simulink model "Irrigation_Control_System_R2020a"  (R2023b)
settings: Solver=VariableStepAuto  StartTime=0.0  StopTime=10.0  MaxStep=1e-3  RelTol=1e-3
libraries: simulink x1
settings Model: Creator=hp  LastModifiedBy=hp
settings SolverCC: AlgebraicLoopSolver=TrustRegion

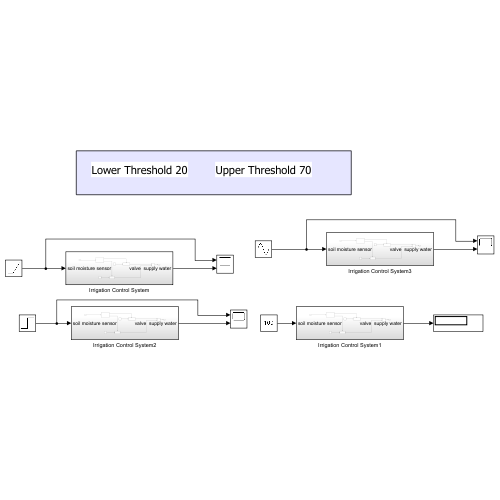
[thumbnail: Simulink's stored preview of the top-level diagram]
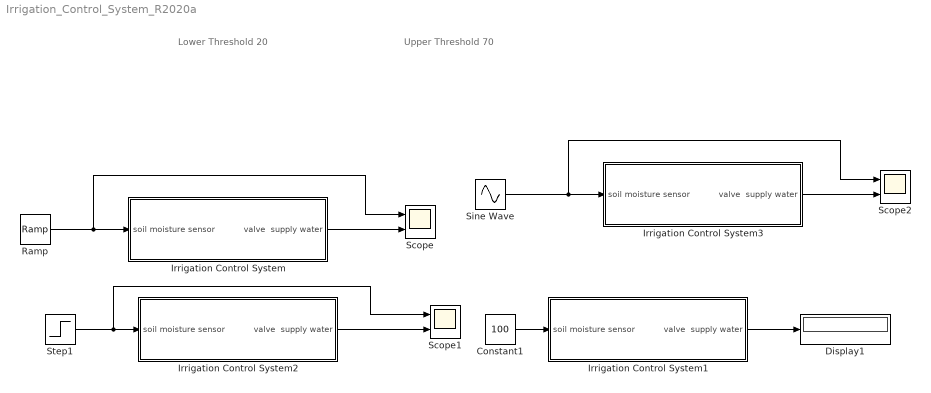
== system Irrigation_Control_System_R2020a ==
  note: Lower Threshold 20
  note: Upper Threshold 70
  Constant1 : Constant  Value=100
  Display1 : Display
  Irrigation Control System : Subsystem
  Irrigation Control System1 : Subsystem
  Irrigation Control System2 : Subsystem
  Irrigation Control System3 : Subsystem
  Ramp : simulink/Sources/Ramp  slope=1  start=0  InitialOutput=15
  Scope : Scope  NumInputPorts=2
  Scope1 : Scope  NumInputPorts=2
  Scope2 : Scope  NumInputPorts=2
  Sine Wave : Sin  Amplitude=50  SampleTime=0
  Step1 : Step  Before=5  After=70  SampleTime=0
  wires:
  Irrigation Control System1/1(valve  supply water) -> Display1/1
  Constant1/1 -> Irrigation Control System1/1(soil moisture sensor)
  Irrigation Control System/1(valve  supply water) -> Scope/2
  Ramp/1 -> Scope/1, Irrigation Control System/1(soil moisture sensor)
  Step1/1 -> Scope1/1, Irrigation Control System2/1(soil moisture sensor)
  Irrigation Control System2/1(valve  supply water) -> Scope1/2
  Sine Wave/1 -> Irrigation Control System3/1(soil moisture sensor), Scope2/1
  Irrigation Control System3/1(valve  supply water) -> Scope2/2

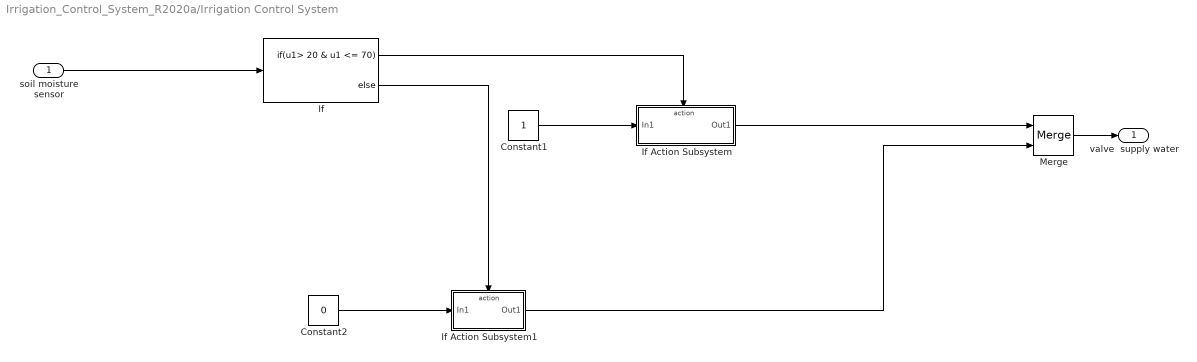
== system Irrigation_Control_System_R2020a/Irrigation Control System ==
  soil moisture sensor : Inport
  Constant1 : Constant
  Constant2 : Constant  Value=0
  If : If  IfExpression=u1> 20 & u1 <= 70
  If Action Subsystem : Subsystem  TreatAsAtomicUnit=on
  If Action Subsystem1 : Subsystem  TreatAsAtomicUnit=on
  Merge : Merge
  valve  supply water : Outport
  wires:
  If Action Subsystem/1(Out1) -> Merge/1
  Constant2/1 -> If Action Subsystem1/1(In1)
  If/2 -> If Action Subsystem1/Action
  If/1 -> If Action Subsystem/Action
  soil moisture sensor/1 -> If/1
  Merge/1 -> valve  supply water/1
  Constant1/1 -> If Action Subsystem/1(In1)
  If Action Subsystem1/1(Out1) -> Merge/2

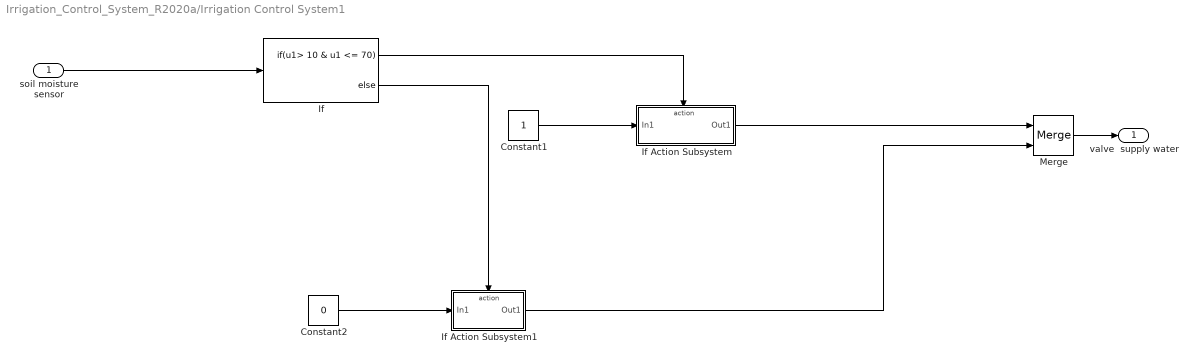
== system Irrigation_Control_System_R2020a/Irrigation Control System1 ==
  soil moisture sensor : Inport
  Constant1 : Constant
  Constant2 : Constant  Value=0
  If : If  IfExpression=u1> 10 & u1 <= 70
  If Action Subsystem : Subsystem  TreatAsAtomicUnit=on
  If Action Subsystem1 : Subsystem  TreatAsAtomicUnit=on
  Merge : Merge
  valve  supply water : Outport
  wires:
  If Action Subsystem1/1(Out1) -> Merge/2
  Constant1/1 -> If Action Subsystem/1(In1)
  Merge/1 -> valve  supply water/1
  soil moisture sensor/1 -> If/1
  If/1 -> If Action Subsystem/Action
  If/2 -> If Action Subsystem1/Action
  Constant2/1 -> If Action Subsystem1/1(In1)
  If Action Subsystem/1(Out1) -> Merge/1

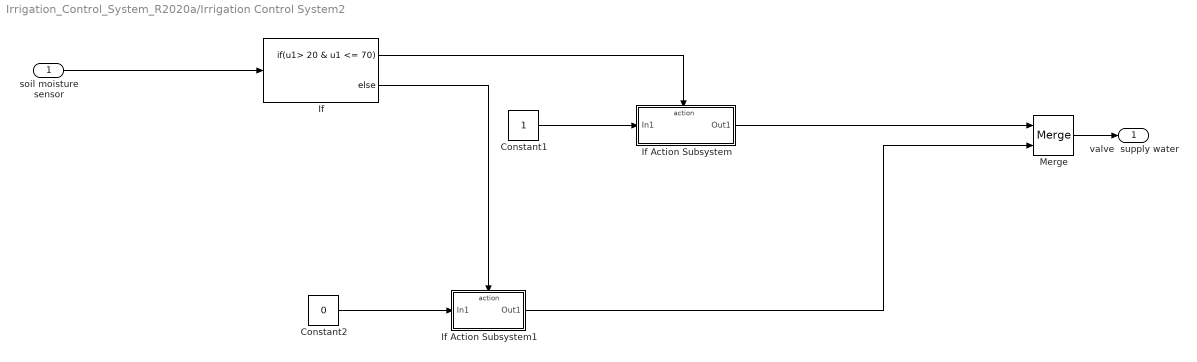
== system Irrigation_Control_System_R2020a/Irrigation Control System2 ==
  soil moisture sensor : Inport
  Constant1 : Constant
  Constant2 : Constant  Value=0
  If : If  IfExpression=u1> 20 & u1 <= 70
  If Action Subsystem : Subsystem  TreatAsAtomicUnit=on
  If Action Subsystem1 : Subsystem  TreatAsAtomicUnit=on
  Merge : Merge
  valve  supply water : Outport
  wires:
  If Action Subsystem1/1(Out1) -> Merge/2
  Constant1/1 -> If Action Subsystem/1(In1)
  Merge/1 -> valve  supply water/1
  soil moisture sensor/1 -> If/1
  If/1 -> If Action Subsystem/Action
  If/2 -> If Action Subsystem1/Action
  Constant2/1 -> If Action Subsystem1/1(In1)
  If Action Subsystem/1(Out1) -> Merge/1

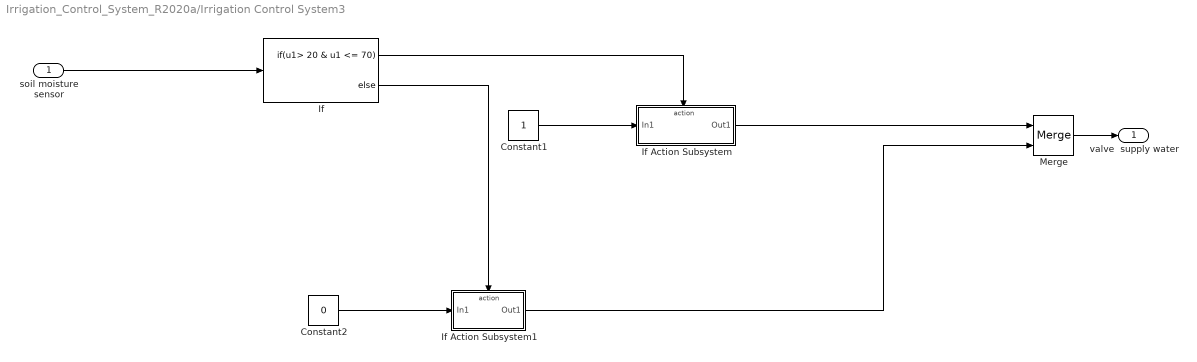
== system Irrigation_Control_System_R2020a/Irrigation Control System3 ==
  soil moisture sensor : Inport
  Constant1 : Constant
  Constant2 : Constant  Value=0
  If : If  IfExpression=u1> 20 & u1 <= 70
  If Action Subsystem : Subsystem  TreatAsAtomicUnit=on
  If Action Subsystem1 : Subsystem  TreatAsAtomicUnit=on
  Merge : Merge
  valve  supply water : Outport
  wires:
  If Action Subsystem1/1(Out1) -> Merge/2
  Constant1/1 -> If Action Subsystem/1(In1)
  Merge/1 -> valve  supply water/1
  soil moisture sensor/1 -> If/1
  If/1 -> If Action Subsystem/Action
  If/2 -> If Action Subsystem1/Action
  Constant2/1 -> If Action Subsystem1/1(In1)
  If Action Subsystem/1(Out1) -> Merge/1

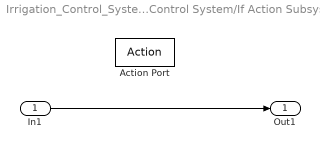
== system Irrigation_Control_System_R2020a/Irrigation Control System/If Action Subsystem ==
  In1 : Inport
  Action Port : ActionPort  ActionPortLabel=if(u1> 20 & u1 <= 70)
  Out1 : Outport
  wires:
  In1/1 -> Out1/1

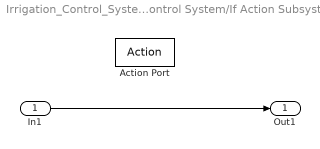
== system Irrigation_Control_System_R2020a/Irrigation Control System/If Action Subsystem1 ==
  In1 : Inport
  Action Port : ActionPort  ActionPortLabel=else
  Out1 : Outport
  wires:
  In1/1 -> Out1/1

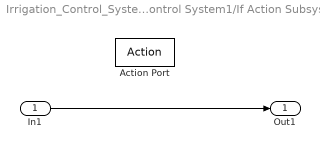
== system Irrigation_Control_System_R2020a/Irrigation Control System1/If Action Subsystem ==
  In1 : Inport
  Action Port : ActionPort  ActionPortLabel=if(u1> 10 & u1 <= 70)
  Out1 : Outport
  wires:
  In1/1 -> Out1/1

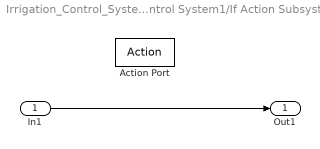
== system Irrigation_Control_System_R2020a/Irrigation Control System1/If Action Subsystem1 ==
  In1 : Inport
  Action Port : ActionPort  ActionPortLabel=else
  Out1 : Outport
  wires:
  In1/1 -> Out1/1

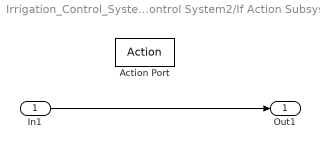
== system Irrigation_Control_System_R2020a/Irrigation Control System2/If Action Subsystem ==
  In1 : Inport
  Action Port : ActionPort  ActionPortLabel=if(u1> 20 & u1 <= 70)
  Out1 : Outport
  wires:
  In1/1 -> Out1/1

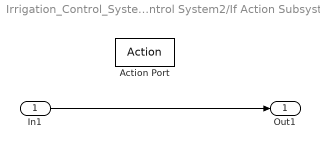
== system Irrigation_Control_System_R2020a/Irrigation Control System2/If Action Subsystem1 ==
  In1 : Inport
  Action Port : ActionPort  ActionPortLabel=else
  Out1 : Outport
  wires:
  In1/1 -> Out1/1

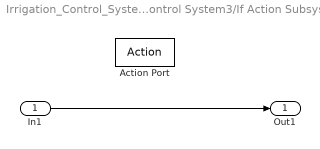
== system Irrigation_Control_System_R2020a/Irrigation Control System3/If Action Subsystem ==
  In1 : Inport
  Action Port : ActionPort  ActionPortLabel=if(u1> 20 & u1 <= 70)
  Out1 : Outport
  wires:
  In1/1 -> Out1/1

== system Irrigation_Control_System_R2020a/Irrigation Control System3/If Action Subsystem1 ==
  In1 : Inport
  Action Port : ActionPort  ActionPortLabel=else
  Out1 : Outport
  wires:
  In1/1 -> Out1/1
